simulink model "roboterrestreESC2014aslx"  (R2015a)
settings: Solver=ode1  StartTime=0.0  StopTime=Tsimu  FixedStep=passo  RelTol=1e-3
values from neighbouring files (symbols this model uses):
  h = (v/Rr)/5    (= 0.314159265359)    [initroboterrestreESC.m]
  Kesc = 0.08    [initroboterrestreESC.m]
  N = 10    [initroboterrestreESC.m]
  Rr = 2    [initroboterrestreESC.m]
  v = 1*pi*Rr/2    (= 3.14159265359)    [initroboterrestreESC.m]
  x0 = zeros(1,5)'    [initroboterrestreESC.m]
libraries: simulink x1
settings Model: CovModelRefEnable=off  Creator=alessandropeixoto  LastModifiedBy=Jean
settings DataIOCC: SaveFormat=StructureWithTime
settings HardwareCC: ProdBitPerPointer=64  ProdLargestAtomicFloat=Float  ProdIntDivRoundTo=Zero  ProdEndianess=LittleEndian  ProdHWDeviceType=Specified
settings GRTTargetCC: GeneratePreprocessorConditionals=Use local settings

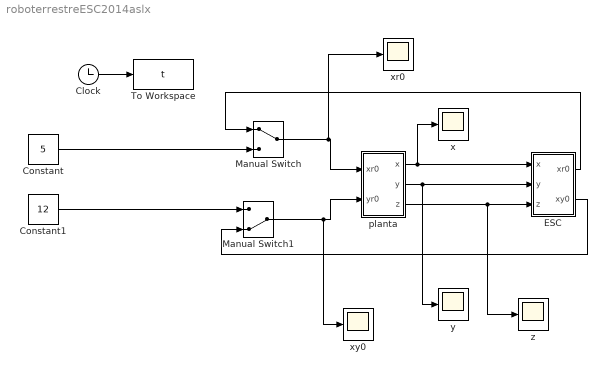
== system roboterrestreESC2014aslx ==
  Clock : Clock
  Constant : Constant  Value=5
  Constant1 : Constant  Value=12
  ESC : Subsystem
  Manual Switch : ManualSwitch
  Manual Switch1 : ManualSwitch  CurrentSetting=0
  To Workspace : ToWorkspace  VariableName=t  SampleTime=-1
  planta : Subsystem
  x : Scope
      settings: YMax=20  SaveName=x
  xr0 : Scope
      settings: YMin=0  YMax=18  SaveName=xrefesc
  xy0 : Scope
      settings: YMin=-6.67587  YMax=17.18725  SaveName=yrefesc
  "y " : Scope
      settings: YMin=-20  SaveName=y
  z : Scope
      settings: TimeRange=40000  YMin=25  YMax=375  SaveName=z
  wires:
  planta/1(x) -> x/1, ESC/1(x)
  planta/2(y) -> "y "/1, ESC/2(y)
  planta/3(z) -> z/1, ESC/3(z)
  Manual Switch/1 -> xr0/1, planta/1(xr0)
  Constant/1 -> Manual Switch/2
  ESC/1(xr0) -> Manual Switch/1
  Constant1/1 -> Manual Switch1/1
  ESC/2(xy0) -> Manual Switch1/2
  Manual Switch1/1 -> xy0/1, planta/2(yr0)
  Clock/1 -> To Workspace/1

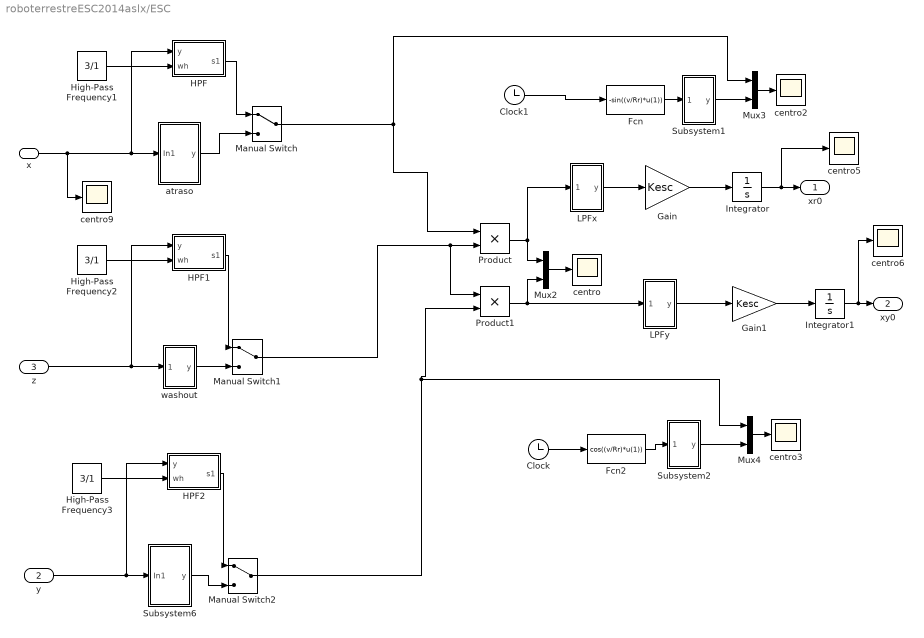
== system roboterrestreESC2014aslx/ESC ==
  x : Inport
  y : Inport  Port=2
  z : Inport  Port=3
  Clock : Clock
  Clock1 : Clock
  Fcn : Fcn  Expr=-sin((v/Rr)*u(1))
  Fcn2 : Fcn  Expr=cos((v/Rr)*u(1))
  Gain : Gain  Gain=Kesc
  Gain1 : Gain  Gain=Kesc
  HPF : Subsystem
  HPF1 : Subsystem
  HPF2 : Subsystem
  High-Pass Frequency1 : Constant  Value=3/1  SampleTime=Inf
  High-Pass Frequency2 : Constant  Value=3/1  SampleTime=Inf
  High-Pass Frequency3 : Constant  Value=3/1  SampleTime=Inf
  Integrator : Integrator  InitialCondition=1
  Integrator1 : Integrator  InitialCondition=1
  LPFx : Subsystem
  LPFy : Subsystem
  Manual Switch : ManualSwitch
  Manual Switch1 : ManualSwitch
  Manual Switch2 : ManualSwitch
  Mux2 : Mux  Inputs=2
  Mux3 : Mux  Inputs=2
  Mux4 : Mux  Inputs=2
  Product : Product
  Product1 : Product
  Subsystem1 : Subsystem
  Subsystem2 : Subsystem
  Subsystem6 : Subsystem
  atraso : Subsystem
  centro{,2..3,5..6,9} (6 alike) : Scope
      centro settings: YMin=-0.52949  YMax=0.71626  SaveName=ScopeData7
      centro2 settings: YMin=-0.23524  YMax=0.25005  SaveName=ScopeData4
      centro3 settings: YMin=-0.22906  YMax=0.2396  SaveName=ScopeData5
      centro5 settings: YMin=-0.23524  YMax=0.25005  SaveName=ScopeData9
      centro6 settings: YMin=-0.23524  YMax=0.25005  SaveName=ScopeData10
      centro9 settings: TimeRange=728.27  YMin=-0.06  YMax=0.04000000000000001  SaveName=xRobot3
  washout : Subsystem
  xr0 : Outport
  xy0 : Outport  Port=2
  wires:
  Manual Switch2/1 -> Product1/2, Mux4/1
  Gain/1 -> Integrator/1
  LPFy/1(y) -> Gain1/1
  x/1 -> centro9/1, HPF/1(y), atraso/1(In1)
  Mux4/1 -> centro3/1
  Integrator1/1 -> centro6/1, xy0/1
  Integrator/1 -> centro5/1, xr0/1
  Manual Switch/1 -> Mux3/1, Product/1
  Product1/1 -> Mux2/2, LPFy/1(In1)
  Subsystem1/1(y) -> Mux3/2
  Subsystem2/1(y) -> Mux4/2
  Mux3/1 -> centro2/1
  Fcn/1 -> Subsystem1/1(In1)
  Fcn2/1 -> Subsystem2/1(In1)
  Clock/1 -> Fcn2/1
  Clock1/1 -> Fcn/1
  Manual Switch1/1 -> Product1/1, Product/2
  Mux2/1 -> centro/1
  Product/1 -> Mux2/1, LPFx/1(In1)
  LPFx/1(y) -> Gain/1
  atraso/1(y) -> Manual Switch/2
  High-Pass Frequency1/1 -> HPF/2(wh)
  HPF/1(s1) -> Manual Switch/1
  z/1 -> HPF1/1(y), washout/1(In1)
  High-Pass Frequency2/1 -> HPF1/2(wh)
  HPF1/1(s1) -> Manual Switch1/1
  y/1 -> HPF2/1(y), Subsystem6/1(In1)
  High-Pass Frequency3/1 -> HPF2/2(wh)
  HPF2/1(s1) -> Manual Switch2/1
  Subsystem6/1(y) -> Manual Switch2/2
  washout/1(y) -> Manual Switch1/2
  Gain1/1 -> Integrator1/1

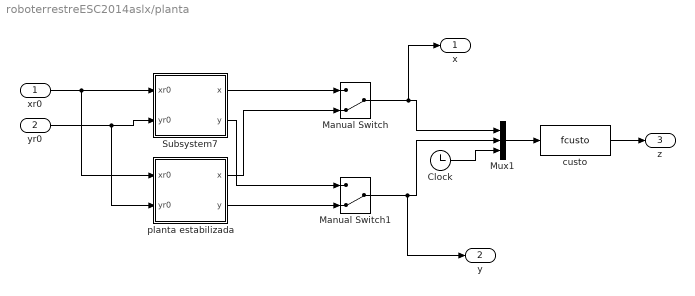
== system roboterrestreESC2014aslx/planta ==
  xr0 : Inport
  yr0 : Inport  Port=2
  Clock : Clock
  Manual Switch : ManualSwitch  CurrentSetting=0
  Manual Switch1 : ManualSwitch  CurrentSetting=0
  Mux1 : Mux  Inputs=3
  Subsystem7 : Subsystem
  custo : MATLABFcn  MATLABFcn=fcusto
  planta estabilizada : Subsystem
  x : Outport
  y : Outport  Port=2
  z : Outport  Port=3
  wires:
  Manual Switch1/1 -> y/1, Mux1/2
  xr0/1 -> planta estabilizada/1(xr0), Subsystem7/1(xr0)
  yr0/1 -> planta estabilizada/2(yr0), Subsystem7/2("yr0 ")
  planta estabilizada/1(x) -> Manual Switch/2
  custo/1 -> z/1
  Manual Switch/1 -> x/1, Mux1/1
  planta estabilizada/2(y) -> Manual Switch1/2
  Subsystem7/2(y) -> Manual Switch1/1
  Mux1/1 -> custo/1
  Subsystem7/1(x) -> Manual Switch/1
  Clock/1 -> Mux1/3

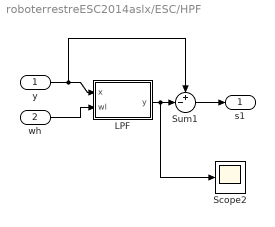
== system roboterrestreESC2014aslx/ESC/HPF ==
  y : Inport
  wh : Inport  Port=2
  LPF : Subsystem
  Scope2 : Scope
      settings: YMin=0.6  YMax=1.125  SaveName=ScopeData5
  Sum1 : Sum  Inputs=+-|
  s1 : Outport
  wires:
  LPF/1(y) -> Sum1/2, Scope2/1
  wh/1 -> LPF/2(wl)
  Sum1/1 -> s1/1
  y/1 -> Sum1/1, LPF/1(x)

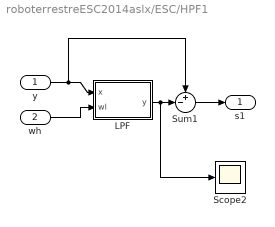
== system roboterrestreESC2014aslx/ESC/HPF1 ==
  y : Inport
  wh : Inport  Port=2
  LPF : Subsystem
  Scope2 : Scope
      settings: YMin=0.6  YMax=1.125  SaveName=ScopeData5
  Sum1 : Sum  Inputs=+-|
  s1 : Outport
  wires:
  y/1 -> LPF/1(x), Sum1/1
  Sum1/1 -> s1/1
  wh/1 -> LPF/2(wl)
  LPF/1(y) -> Scope2/1, Sum1/2

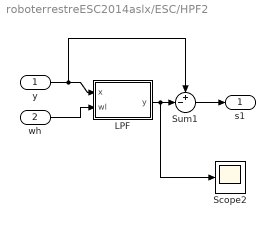
== system roboterrestreESC2014aslx/ESC/HPF2 ==
  y : Inport
  wh : Inport  Port=2
  LPF : Subsystem
  Scope2 : Scope
      settings: YMin=0.6  YMax=1.125  SaveName=ScopeData5
  Sum1 : Sum  Inputs=+-|
  s1 : Outport
  wires:
  y/1 -> LPF/1(x), Sum1/1
  Sum1/1 -> s1/1
  wh/1 -> LPF/2(wl)
  LPF/1(y) -> Scope2/1, Sum1/2

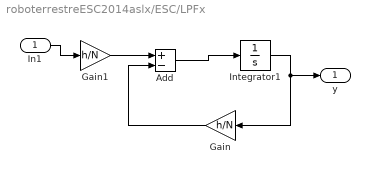
== system roboterrestreESC2014aslx/ESC/LPFx ==
  In1 : Inport
  Add : Sum  Inputs=+-
  Gain : Gain  Gain=h/N
  Gain1 : Gain  Gain=h/N
  Integrator1 : Integrator
  y : Outport
  wires:
  Add/1 -> Integrator1/1
  In1/1 -> Gain1/1
  Gain/1 -> Add/2
  Integrator1/1 -> y/1, Gain/1
  Gain1/1 -> Add/1

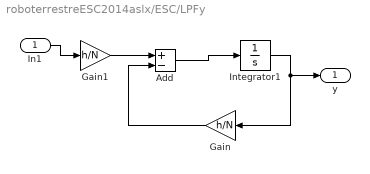
== system roboterrestreESC2014aslx/ESC/LPFy ==
  In1 : Inport
  Add : Sum  Inputs=+-
  Gain : Gain  Gain=h/N
  Gain1 : Gain  Gain=h/N
  Integrator1 : Integrator
  y : Outport
  wires:
  Add/1 -> Integrator1/1
  In1/1 -> Gain1/1
  Gain/1 -> Add/2
  Integrator1/1 -> y/1, Gain/1
  Gain1/1 -> Add/1

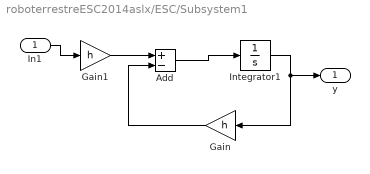
== system roboterrestreESC2014aslx/ESC/Subsystem1 ==
  In1 : Inport
  Add : Sum  Inputs=+-
  Gain : Gain  Gain=h
  Gain1 : Gain  Gain=h
  Integrator1 : Integrator
  y : Outport
  wires:
  Add/1 -> Integrator1/1
  In1/1 -> Gain1/1
  Gain/1 -> Add/2
  Integrator1/1 -> y/1, Gain/1
  Gain1/1 -> Add/1

== system roboterrestreESC2014aslx/ESC/Subsystem2 ==
  In1 : Inport
  Add : Sum  Inputs=+-
  Gain : Gain  Gain=h
  Gain1 : Gain  Gain=h
  Integrator1 : Integrator
  y : Outport
  wires:
  Add/1 -> Integrator1/1
  In1/1 -> Gain1/1
  Gain/1 -> Add/2
  Integrator1/1 -> y/1, Gain/1
  Gain1/1 -> Add/1

== system roboterrestreESC2014aslx/ESC/Subsystem6 ==
  In1 : Inport
  Add : Sum  Inputs=+-
  Gain : Gain  Gain=h
  Integrator1 : Integrator
  y : Outport
  wires:
  Add/1 -> y/1, Integrator1/1
  Integrator1/1 -> Gain/1
  In1/1 -> Add/1
  Gain/1 -> Add/2

== system roboterrestreESC2014aslx/ESC/atraso ==
  In1 : Inport
  Add : Sum  Inputs=+-
  Gain : Gain  Gain=h
  Integrator1 : Integrator
  y : Outport
  wires:
  Add/1 -> y/1, Integrator1/1
  Integrator1/1 -> Gain/1
  In1/1 -> Add/1
  Gain/1 -> Add/2

== system roboterrestreESC2014aslx/ESC/washout ==
  In1 : Inport
  Add : Sum  Inputs=+-
  Gain : Gain  Gain=h
  Integrator1 : Integrator
  y : Outport
  wires:
  Add/1 -> y/1, Integrator1/1
  Integrator1/1 -> Gain/1
  In1/1 -> Add/1
  Gain/1 -> Add/2

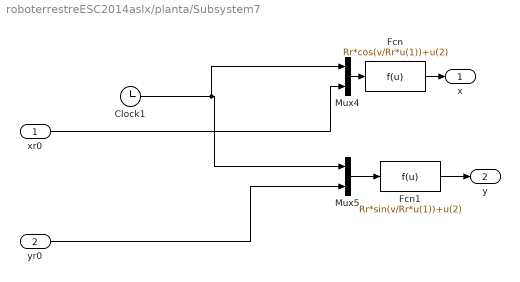
== system roboterrestreESC2014aslx/planta/Subsystem7 ==
  xr0 : Inport
  "yr0 " : Inport  Port=2
  Clock1 : Clock
  Fcn : Fcn  Expr=Rr*cos(v/Rr*u(1))+u(2)
  Fcn1 : Fcn  Expr=Rr*sin(v/Rr*u(1))+u(2)
  Mux4 : Mux  Inputs=2
  Mux5 : Mux  Inputs=2
  x : Outport
  y : Outport  Port=2
  wires:
  xr0/1 -> Mux4/2
  Mux5/1 -> Fcn1/1
  Fcn1/1 -> y/1
  Mux4/1 -> Fcn/1
  Clock1/1 -> Mux5/1, Mux4/1
  "yr0 "/1 -> Mux5/2
  Fcn/1 -> x/1

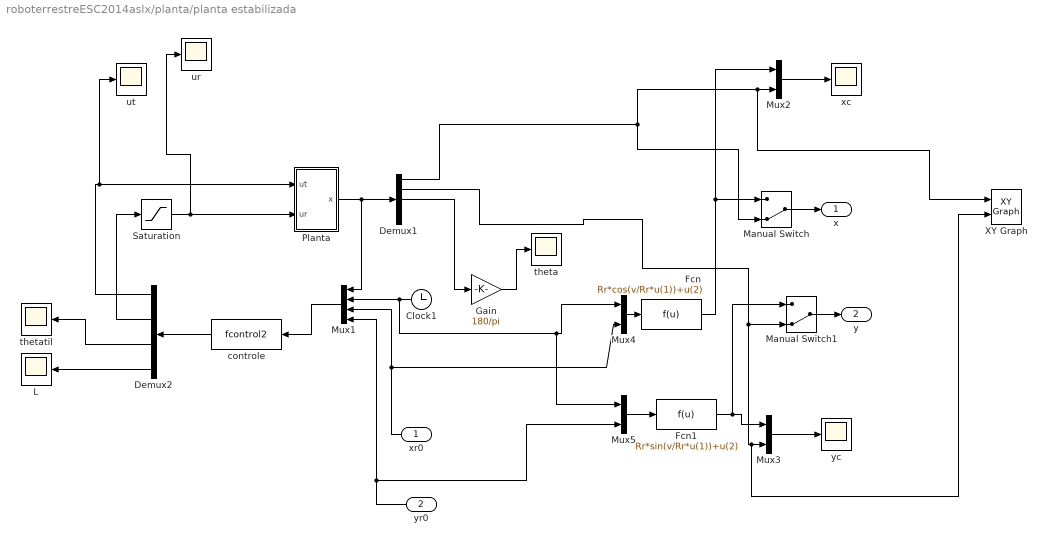
== system roboterrestreESC2014aslx/planta/planta estabilizada ==
  xr0 : Inport
  yr0 : Inport  Port=2
  Clock1 : Clock
  Demux1 : Demux  Outputs=5
  Demux2 : Demux
  Fcn : Fcn  Expr=Rr*cos(v/Rr*u(1))+u(2)
  Fcn1 : Fcn  Expr=Rr*sin(v/Rr*u(1))+u(2)
  Gain : Gain  Gain=180/pi
  L : Scope
      settings: YMin=-0.16559  YMax=1.54394  SaveName=ScopeData6
  Manual Switch : ManualSwitch  CurrentSetting=0
  Manual Switch1 : ManualSwitch  CurrentSetting=0
  Mux1 : Mux
  Mux{2..5} (4 alike) : Mux  Inputs=2
  Planta : Subsystem
  Saturation : Saturate  UpperLimit=10  LowerLimit=-10
  XY Graph : simulink/Sinks/XY Graph  xmin=-50  xmax=50  ymin=-50  ymax=50  st=-1
  controle : MATLABFcn  MATLABFcn=fcontrol2
  theta : Scope
      settings: YMin=-315507.35399  YMax=35056.37267  SaveName=ScopeData4
  thetatil : Scope
      settings: YMin=-7370.79779  YMax=59109.94409  SaveName=ScopeData5
  ur : Scope
      settings: YMin=-315507.35399  YMax=35056.37267  SaveName=ur
  ut : Scope
      settings: YMin=-315507.35399  YMax=35056.37267  SaveName=ut
  xc : Scope
      settings: YMin=53.25  YMax=58.5
  yc : Scope
      settings: YMin=0.82677  YMax=1.1445  SaveName=ScopeData2
  x : Outport
  y : Outport  Port=2
  wires:
  Demux1/1 -> Manual Switch/2, XY Graph/1, Mux2/2
  controle/1 -> Demux2/1
  Planta/1(x) -> Demux1/1, Mux1/1
  Clock1/1 -> Mux5/1, Mux4/1, Mux1/2
  Demux1/3 -> Gain/1
  Demux2/2 -> Saturation/1
  yr0/1 -> Mux5/2, Mux1/4
  Gain/1 -> theta/1
  Demux2/4 -> L/1
  Mux1/1 -> controle/1
  Demux2/3 -> thetatil/1
  Demux2/1 -> ut/1, Planta/1(ut)
  xr0/1 -> Mux1/3, Mux4/2
  Mux2/1 -> xc/1
  Fcn/1 -> Manual Switch/1, Mux2/1
  Mux3/1 -> yc/1
  Fcn1/1 -> Manual Switch1/1, Mux3/1
  Mux4/1 -> Fcn/1
  Mux5/1 -> Fcn1/1
  Demux1/2 -> XY Graph/2, Mux3/2, Manual Switch1/2
  Manual Switch/1 -> x/1
  Manual Switch1/1 -> y/1
  Saturation/1 -> Planta/2(ur), ur/1

== system roboterrestreESC2014aslx/ESC/HPF/LPF ==
  x : Inport
  wl : Inport  Port=2
  Integrator : Integrator
  Product2 : Product
  Sum : Sum  Inputs=|+-
  y : Outport
  wires:
  wl/1 -> Product2/1
  Integrator/1 -> y/1, Sum/2
  Product2/1 -> Integrator/1
  Sum/1 -> Product2/2
  x/1 -> Sum/1

== system roboterrestreESC2014aslx/ESC/HPF1/LPF ==
  x : Inport
  wl : Inport  Port=2
  Integrator : Integrator
  Product2 : Product
  Sum : Sum  Inputs=|+-
  y : Outport
  wires:
  x/1 -> Sum/1
  Sum/1 -> Product2/2
  Product2/1 -> Integrator/1
  Integrator/1 -> Sum/2, y/1
  wl/1 -> Product2/1

== system roboterrestreESC2014aslx/ESC/HPF2/LPF ==
  x : Inport
  wl : Inport  Port=2
  Integrator : Integrator
  Product2 : Product
  Sum : Sum  Inputs=|+-
  y : Outport
  wires:
  x/1 -> Sum/1
  Sum/1 -> Product2/2
  Product2/1 -> Integrator/1
  Integrator/1 -> Sum/2, y/1
  wl/1 -> Product2/1

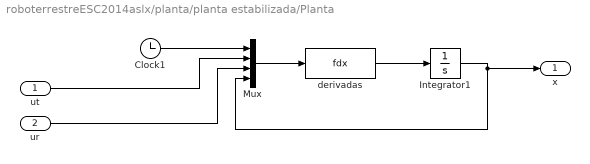
== system roboterrestreESC2014aslx/planta/planta estabilizada/Planta ==
  ut : Inport
  ur : Inport  Port=2
  Clock1 : Clock
  Integrator1 : Integrator  InitialCondition=x0
  Mux : Mux
  derivadas : MATLABFcn  MATLABFcn=fdx
  x : Outport
  wires:
  ur/1 -> Mux/3
  ut/1 -> Mux/2
  Clock1/1 -> Mux/1
  Mux/1 -> derivadas/1
  Integrator1/1 -> x/1, Mux/4
  derivadas/1 -> Integrator1/1
